simulink model "p1sim"  (R2021a)
settings: Solver=ode45  StartTime=0.0  StopTime=100  RelTol=1e-10
values from neighbouring files (symbols this model uses):
  g = 9.81    [alg1.m]    (also in alg2.m; edda-ctc-script.m; edda-pd-script.m)
  Kd = 10000    [alg1.m]    (also in edda-pd-script.m)
  Kp = 100000    [alg1.m]    (also in edda-pd-script.m)
  Theta1 = 3.1    [alg1.m]    (also in alg2.m; edda-ctc-script.m; edda-pd-script.m)
  Theta2 = 9.5    [alg1.m]    (also in alg2.m; edda-ctc-script.m; edda-pd-script.m)
  Theta3 = 0.24    [alg1.m]    (also in alg2.m; edda-ctc-script.m; edda-pd-script.m)
  Theta4 = 0.77    [alg1.m]    (also in alg2.m; edda-ctc-script.m; edda-pd-script.m)
settings Model: Creator=lajk0  LastModifiedBy=kacpe
settings DataIOCC: ReturnWorkspaceOutputs=off

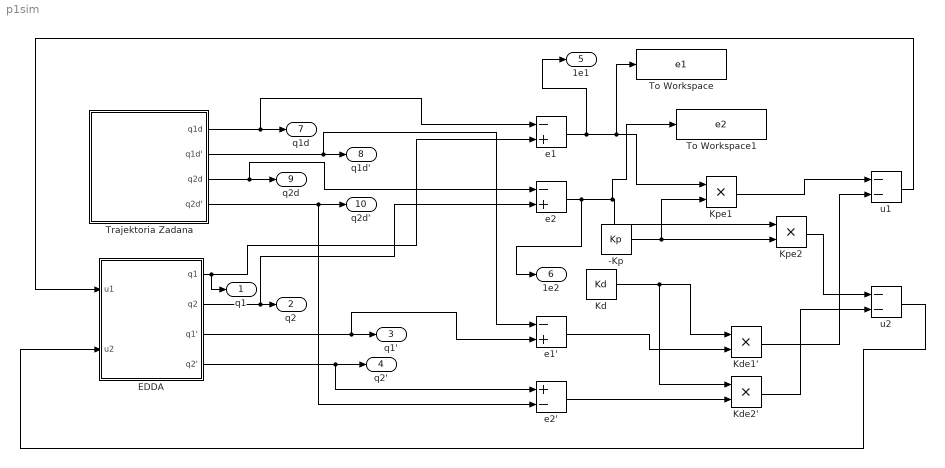
== system p1sim ==
  " u1" : Sum  Inputs=--
  " u2" : Sum  Inputs=--
  -Kp : Constant  Value=Kp
  EDDA : Subsystem
  Kd : Constant  Value=Kd
  Kde1' : Product
  Kde2' : Product
  Kpe1 : Product
  Kpe2 : Product
  To Workspace : ToWorkspace  VariableName=e1  SampleTime=-1
  To Workspace1 : ToWorkspace  VariableName=e2  SampleTime=-1
  Trajektoria Zadana : Subsystem
  e1 : Sum  Inputs=-+
  e1' : Sum  Inputs=-+
  e2 : Sum  Inputs=-+
  e2' : Sum  Inputs=+-
  q1 : Outport
  q2 : Outport  Port=2
  q1' : Outport  Port=3
  q2' : Outport  Port=4
  1e1 : Outport  Port=5
  1e2 : Outport  Port=6
  q1d : Outport  Port=7
  q1d' : Outport  Port=8
  q2d : Outport  Port=9
  q2d' : Outport  Port=10
  wires:
  " u2"/1 -> EDDA/2(u2)
  " u1"/1 -> EDDA/1(u1)
  EDDA/3(q1') -> e1'/2, q1'/1
  EDDA/4(q2') -> e2'/1, q2'/1
  EDDA/1(q1) -> e1/2, q1/1
  EDDA/2(q2) -> e2/2, q2/1
  Trajektoria Zadana/1(q1d) -> q1d/1, e1/1
  Trajektoria Zadana/2(q1d') -> q1d'/1, e1'/1
  Trajektoria Zadana/3(q2d) -> q2d/1, e2/1
  Trajektoria Zadana/4(q2d') -> q2d'/1, e2'/2
  e1/1 -> 1e1/1, To Workspace/1, Kpe1/1
  -Kp/1 -> Kpe2/2, Kpe1/2
  e2/1 -> 1e2/1, To Workspace1/1, Kpe2/1
  e1'/1 -> Kde1'/2
  e2'/1 -> Kde2'/2
  Kd/1 -> Kde2'/1, Kde1'/1
  Kde1'/1 -> " u1"/2
  Kpe1/1 -> " u1"/1
  Kpe2/1 -> " u2"/1
  Kde2'/1 -> " u2"/2

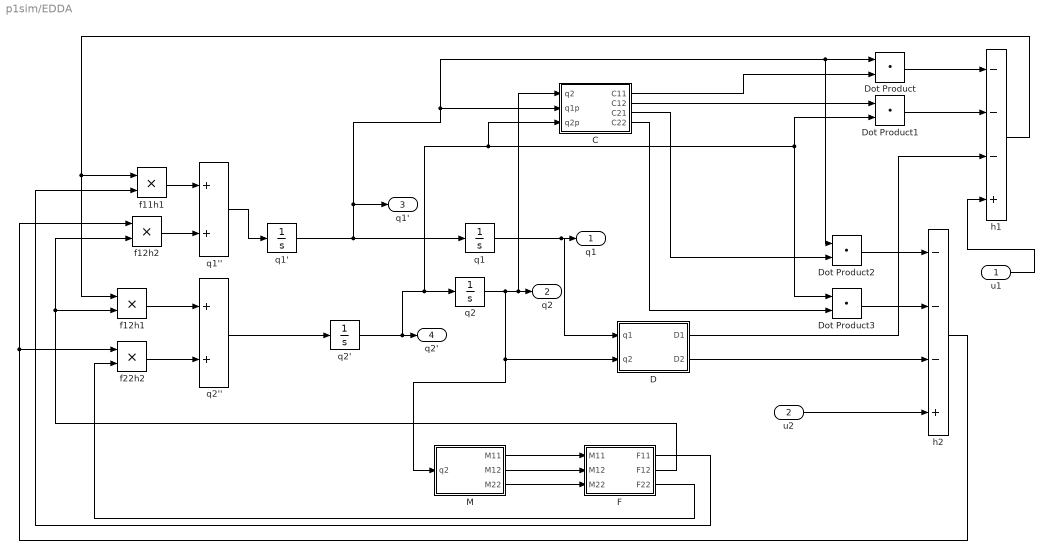
== system p1sim/EDDA ==
  u1 : Inport
  u2 : Inport  Port=2
  " q1" : Integrator
  " q1'" : Integrator
  " q2" : Integrator
  " q2'" : Integrator
  C : MATLAB Function  TreatAsAtomicUnit=on
  D : MATLAB Function  TreatAsAtomicUnit=on
  Dot Product{,1..3} (4 alike) : DotProduct  InputSameDT=on  OutDataTypeStr=Inherit: Inherit via internal rule
  F : MATLAB Function  TreatAsAtomicUnit=on
  M : MATLAB Function  TreatAsAtomicUnit=on
  f11h1 : Product
  f12h1 : Product
  f12h2 : Product
  f22h2 : Product
  h1 : Sum  Inputs=---+
  h2 : Sum  Inputs=---+
  q1'' : Sum
  q2'' : Sum
  q1 : Outport
  q2 : Outport  Port=2
  q1' : Outport  Port=3
  q2' : Outport  Port=4
  wires:
  u1/1 -> h1/4
  u2/1 -> h2/4
  " q2'"/1 -> C/3(q2p), Dot Product3/1, Dot Product1/2, " q2"/1, q2'/1
  " q2"/1 -> M/1(q2), D/2(q2), q2/1, C/1(q2)
  " q1"/1 -> D/1(q1), q1/1
  M/1(M11) -> F/1(M11)
  M/2(M12) -> F/2(M12)
  M/3(M22) -> F/3(M22)
  Dot Product/1 -> h1/1
  C/1(C11) -> Dot Product/2
  Dot Product1/1 -> h1/2
  C/2(C12) -> Dot Product1/1
  D/1(D1) -> h1/3
  D/2(D2) -> h2/3
  Dot Product2/1 -> h2/1
  Dot Product3/1 -> h2/2
  C/3(C21) -> Dot Product2/2
  C/4(C22) -> Dot Product3/2
  " q1'"/1 -> q1'/1, Dot Product2/1, Dot Product/1, C/2(q1p), " q1"/1
  h1/1 -> f12h1/1, f11h1/1
  F/3(F22) -> f22h2/2
  F/2(F12) -> f12h2/2, f12h1/2
  F/1(F11) -> f11h1/2
  q1''/1 -> " q1'"/1
  q2''/1 -> " q2'"/1
  f11h1/1 -> q1''/1
  f12h2/1 -> q1''/2
  f12h1/1 -> q2''/1
  f22h2/1 -> q2''/2
  h2/1 -> f12h2/1, f22h2/1

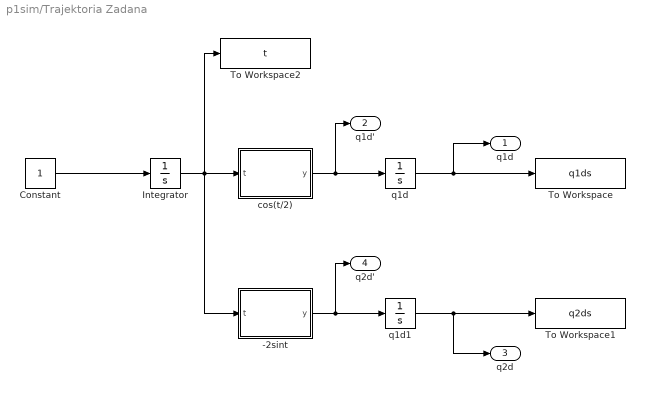
== system p1sim/Trajektoria Zadana ==
  " q1d" : Integrator
  " q1d1" : Integrator  InitialCondition=2
  -2sint : MATLAB Function  TreatAsAtomicUnit=on
  Constant : Constant
  Integrator : Integrator
  To Workspace : ToWorkspace  VariableName=q1ds  SampleTime=-1
  To Workspace1 : ToWorkspace  VariableName=q2ds  SampleTime=-1
  To Workspace2 : ToWorkspace  VariableName=t  SampleTime=-1
  cos(t/2) : MATLAB Function  TreatAsAtomicUnit=on
  q1d : Outport
  q1d' : Outport  Port=2
  q2d : Outport  Port=3
  q2d' : Outport  Port=4
  wires:
  Integrator/1 -> To Workspace2/1, -2sint/1(t), cos(t/2)/1(t)
  Constant/1 -> Integrator/1
  cos(t/2)/1(y) -> q1d'/1, " q1d"/1
  " q1d"/1 -> To Workspace/1, q1d/1
  -2sint/1(y) -> q2d'/1, " q1d1"/1
  " q1d1"/1 -> To Workspace1/1, q2d/1

== matlab function p1sim/EDDA/M ==
  data: q2 input; M11 output; M12 output; M22 output; Theta1 parameter; Theta3 parameter; Theta4 parameter
function [M11, M12,  M22]= fcn(q2, Theta1,  Theta3, Theta4)

M11=Theta1+0.6*Theta4*cos(q2);
M12=Theta3+0.3*Theta4*cos(q2);
%M21=Theta3+0.3*Theta4*cos(q2);
M22=Theta3;

== matlab function p1sim/EDDA/C ==
  data: q2 input; C11 output; q1p input; q2p input; C12 output; C21 output; C22 output; Theta4 parameter
function [C11,C12,C21,C22]= fcn(q2 ,q1p  ,q2p, Theta4)
a=0.3*Theta4*sin(q2);
C11=-q2p*a;
C12=-(q1p+q2p)*a;
C21=q1p*a;
C22=0*a;

== matlab function p1sim/EDDA/D ==
  data: q1 input; D1 output; q2 input; D2 output; g parameter; Theta4 parameter; Theta2 parameter
function [D1, D2]= fcn(q1, q2, g, Theta4, Theta2)

D1=Theta2*cos(q1)+Theta4*cos(q1+q2)*g;
D2=Theta4*cos(q1+q2)*g;

== matlab function p1sim/EDDA/F ==
  data: M11 input; F11 output; M12 input; M22 input; F12 output; F22 output
function [F11, F12,  F22]= fcn(M11, M12,  M22)

Det=M11*M22-M12*M12;
F11=M22/Det;
F12=-M12/Det;
F22=M11/Det;

== matlab function p1sim/Trajektoria Zadana/cos(t//2) ==
  data: t input; y output
function y = fcn(t)

y = cos(t/2);

== matlab function p1sim/Trajektoria Zadana/-2sint ==
  data: t input; y output
function y = fcn(t)

y = -2*sin(t);
